simulink model "Turbine"  (R2022b)
settings: Solver=VariableStepAuto  StartTime=0.0  StopTime=10.0  RelTol=1e-3
settings Model: Creator=Crapon  LastModifiedBy=Crapon

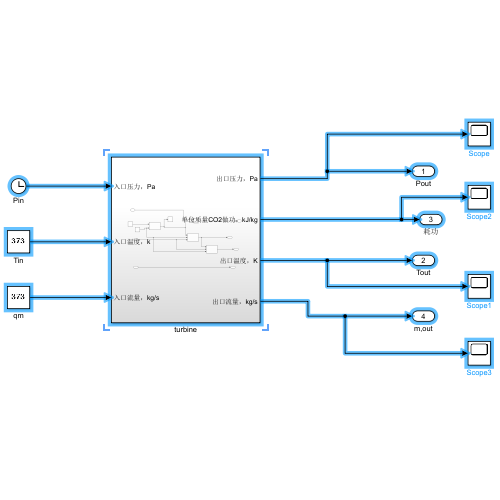
[thumbnail: Simulink's stored preview of the top-level diagram]
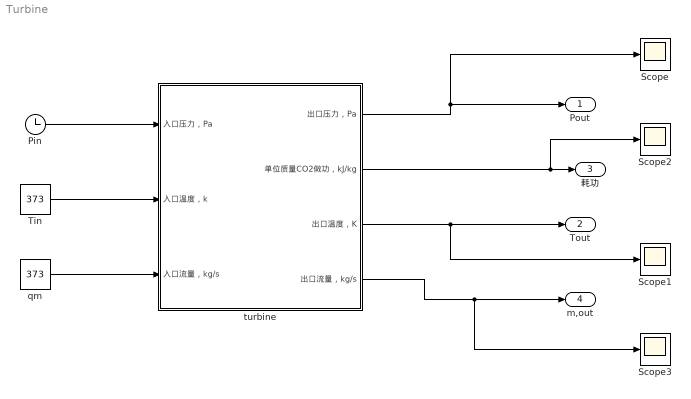
== system Turbine ==
  Pin : Clock
  Scope{,1..3} (4 alike) : Scope
  Tin : Constant  Value=373
  qm : Constant  Value=373
  turbine : Subsystem
  Pout : Outport
  Tout : Outport  Port=2
  耗功 : Outport  Port=3
  m,out : Outport  Port=4
  wires:
  turbine/4("  出口流量，kg/s") -> Scope3/1, m,out/1
  qm/1 -> turbine/3(入口流量，kg/s)
  Pin/1 -> turbine/1(入口压力，Pa)
  turbine/2(单位质量CO2做功，kJ/kg) -> Scope2/1, 耗功/1
  turbine/3(出口温度，K) -> Tout/1, Scope1/1
  Tin/1 -> turbine/2(入口温度，k)
  turbine/1(出口压力，Pa) -> Scope/1, Pout/1

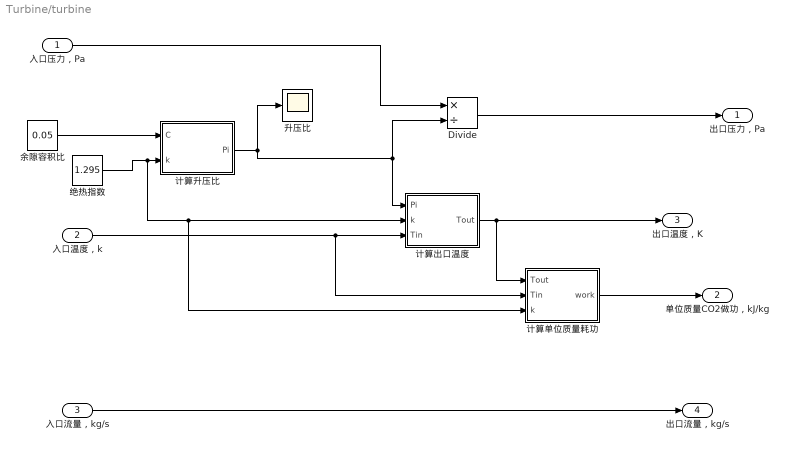
== system Turbine/turbine ==
  入口压力，Pa : Inport
  入口温度，k : Inport  Port=2
  入口流量，kg/s : Inport  Port=3
  Divide : Product  Inputs=*/
  余隙容积比 : Constant  Value=0.05
  升压比 : Scope
  绝热指数 : Constant  Value=1.295
  计算出口温度 : MATLAB Function  TreatAsAtomicUnit=on
  计算升压比 : MATLAB Function  TreatAsAtomicUnit=on
  计算单位质量耗功 : MATLAB Function  TreatAsAtomicUnit=on
  出口压力，Pa : Outport
  单位质量CO2做功，kJ/kg : Outport  Port=2
  出口温度，K : Outport  Port=3
  "  出口流量，kg/s" : Outport  Port=4
  wires:
  余隙容积比/1 -> 计算升压比/1(C)
  入口压力，Pa/1 -> Divide/1
  绝热指数/1 -> 计算单位质量耗功/3(k), 计算出口温度/2(k), 计算升压比/2(k)
  Divide/1 -> 出口压力，Pa/1
  计算单位质量耗功/1(work) -> 单位质量CO2做功，kJ/kg/1
  计算升压比/1(Pi) -> Divide/2, 计算出口温度/1(Pi), 升压比/1
  入口温度，k/1 -> 计算单位质量耗功/2(Tin), 计算出口温度/3(Tin)
  计算出口温度/1(Tout) -> 出口温度，K/1, 计算单位质量耗功/1(Tout)
  入口流量，kg/s/1 -> "  出口流量，kg/s"/1

== matlab function Turbine/turbine/计算出口温度 ==
  data: Pi input; Tout output; k input; Tin input
function Tout= fcn(Pi, k, Tin)

Tout=Tin/((Pi)^((k-1)/k));

== matlab function Turbine/turbine/计算单位质量耗功 ==
  data: Tout input; Tin input; k input; work output
function work= fcn(Tout,Tin,k)
Rg=0.189;
work=(k/(k-1))*Rg*(-Tout+Tin);

== matlab function Turbine/turbine/计算升压比 ==
  data: C input; Pi output; k input
function Pi = fcn(C, k)

Pi =(1+1/C)^k;
